simulink model "math_amp"  (Simulink 6.0)
settings: Solver=ode45  StartTime=0.0  StopTime=10.0  RelTol=1e-3
undefined symbols (not defined in the file or in its folder): dTypeID, Fs
libraries: dspsnks4 x2, rfmathmodels1 x1, dspmtrx3 x1, simulink x1
settings Model: Creator=ashivapr  LastModifiedBy=cvora  ExtModeAutoUpdateStatusClock=off  ProdHWDeviceType=Specified
settings DataIOCC: SaveOutput=off  SaveTime=off  SignalLoggingName=logsOut
settings DebuggingCC: CheckExecutionContextPreStartOutputMsg=on  CheckExecutionContextRuntimeOutputMsg=on  SolverPrmCheckMsg=none
settings HardwareCC: ProdHWDeviceType=Specified
settings ModelReferenceCC: UpdateModelReferenceTargets=IfOutOfDate
settings GRTTargetCC: LifeSpan=inf
settings SFSimCC: SFSimApplyToAllLibs=on  SFSimBuildMode=Incremental

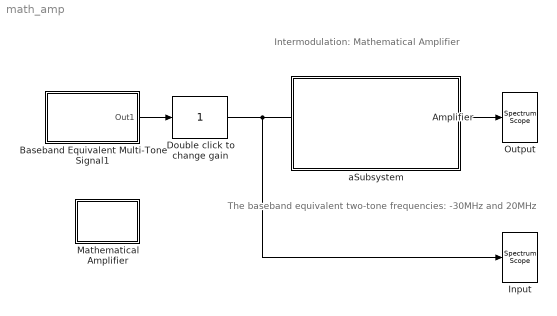
== system math_amp ==
  note: Intermodulation: Mathematical Amplifier
  note: The baseband equivalent
      |  two-tone frequencies:
      | -30MHz and 20MHz
  Amplifier : rfmathmodels1/Amplifier  model_select=Hyperbolic tangent  linGaindB=0  GindB=0  iip3=30  am2pm=0  amam=[2.1587 1.1517]  ampm=[4.0033 9.1040]  x=[8.1081 1.5413 6.5202 -0.0718]  y=[4.6645 2.0965 10.88 -0.003]  p=0.5  GoutdB=0  vsat=1  method_select=Noise figure  ntemp=290  nfigure=3.01  nfactor=2  seed=67987
  Baseband Equivalent Multi-Tone Signal1 : Subsystem  EnableExecutionContextPropagation=on  mask(Baseband Equivalent Multi-Tone Sine Wave){Fc=2.1e9, Frequency=[2.07e9 2.12e9], Amplitude=[0.01 0.005], Phase=[0 pi/4], SampleTime=3e-9, SamplesPerFrame=256}
      mask prompts: Fc "Center frequency (Hz)"; Frequency "Tone frequency (Hz):"; Amplitude "Tone amplitude:"; Phase "Tone phase offset (rad):"; SampleTime "Sample time:"; SamplesPerFrame "Samples per frame:"
      mask help:
      | Generate a baseband equivalent multi-tone complex sinusoid signal. The frequency of the output multi-tone signal is the difference between the Tone frequency and the Center frequency.
      |
      | The values specified here for the Center frequency and Sample time parameters should be equal to the values specified in the 'Input Port' block.
      mask init:
      | if ~isscalar(Fc)
      | 	error('Center frequency must be a scalar');
      | end
      | if ~isnumeric(Frequency)
      | 	error('Tone frequency must be a real vector');
      | end
      | if any(Frequency>=2*Fc)
      | 	error('Tone frequency is too large compared to the Center frequency');
      | end
      | 
      | Frequency = Frequency-Fc;
      mask Display:
      | plot(-0.5,-3,1.5,1,[0:0.005:1], [0.25*sin(2*pi*5*[0:0.005:1])+0.5*sin(2*pi*10*[0:0.005:1]) ]);
      | disp('\nMulti-Tone');
  Double click to change gain : simulink/Math Operations/Slider Gain  low=1  gain=1  high=10
  Input : dspsnks4/Spectrum Scope  ScopeProperties=off  Domain=Frequency  HorizSpan=1  UseBuffer=off  BufferSize=128  Overlap=64  inpFftLenInherit=off  FFTlength=1024  numAvg=20  DisplayProperties=on  AxisGrid=on  Memory=off  FrameNumber=off  AxisLegend=off  AxisZoom=off  OpenScopeAtSimStart=on  OpenScopeImmediately=off  FigPos=[6 311 333 250]  AxisProperties=off  XUnits=Hertz  XRange=[-Fs/2...Fs/2]  InheritXIncr=on  XIncr=1.0  XLabel=Samples  YUnits=dB  YLabel=Magnitude, dB  LineProperties=off
      settings: YMin=-162.913297942411  YMax=-10.4261857162777
  Mathematical Amplifier : Subsystem  EnableExecutionContextPropagation=on
      mask Display: disp('Info')
  Output : dspsnks4/Spectrum Scope  ScopeProperties=off  Domain=Frequency  HorizSpan=1  UseBuffer=off  BufferSize=128  Overlap=64  inpFftLenInherit=off  FFTlength=1024  numAvg=20  DisplayProperties=on  AxisGrid=on  Memory=off  FrameNumber=off  AxisLegend=off  AxisZoom=off  OpenScopeAtSimStart=on  OpenScopeImmediately=off  FigPos=[346 311 350 250]  AxisProperties=off  XUnits=Hertz  XRange=[-Fs/2...Fs/2]  InheritXIncr=on  XIncr=1.0  XLabel=Samples  YUnits=dB  YLabel=Magnitude, dB  LineProperties=off
      settings: YMin=-127.684741352242  YMax=8.6774665535425
  aSubsystem : Subsystem  EnableExecutionContextPropagation=on
      mask Display: disp('')
  wires:
  Baseband Equivalent Multi-Tone Signal1/1(Out1) -> Double click to change gain/1
  Amplifier/1 -> Output/1
  Double click to change gain/1 -> Input/1, Amplifier/1

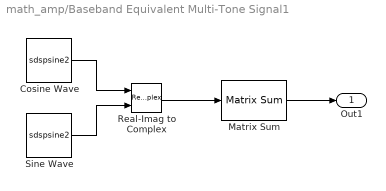
== system math_amp/Baseband Equivalent Multi-Tone Signal1 ==
  Cosine Wave : S-Function  AncestorBlock=dspsrcs4/Sine Wave  FunctionName=sdspsine2  Parameters=Amplitude,Frequency,Phase,SampleMode,OutComplex,CompMethod,SampleTime,SamplesPerFrame,ResetState,TableSize,isCustomFloat,isSigned,dTypeID,wordLength,fracBits  mask(Sine Wave){Amplitude=Amplitude, Frequency=Frequency, Phase=Phase+(pi/2), SampleMode=Discrete, OutComplex=Real, CompMethod=Trigonometric fcn, TableSize=Speed, SampleTime=SampleTime, SamplesPerFrame=SamplesPerFrame, additionalParams=off, allowOverrides=on, dataType=double, wordLen=16, udDataType=sfix(16), fracBitsMode=Best precision, numFracBits=15, ResetState=Restart at time zero}
      mask prompts: Frequency "Frequency (Hz):"; Phase "Phase offset (rad):"; SampleMode "Sample mode:"; OutComplex "Output complexity:"; CompMethod "Computation method:"; TableSize "Optimize table for:"; SampleTime "Sample time:"; SamplesPerFrame "Samples per frame:"; additionalParams "------- Show additional parameters --------"; allowOverrides "Allow overrides from DSP Fixed-Point Attributes blocks"; dataType "Output data type:"; wordLen "Word length:"; udDataType "User-defined data type (e.g. sfix(16), float('single')):"; fracBitsMode "Set fraction length in output to:"; numFracBits "Fraction length:"; ResetState "State when re-enabled:"
      mask help: Output samples of a sinusoid. To generate more than one sinusoid simultaneously, enter a vector of values for the amplitude, frequency, and phase parameters.
      mask init:
      | [x,y] = dspblksine('icon');
      | [dtInfo,dTypeID]=dspblksine('init');
      | isSigned=dtInfo.DataTypeIsSigned;
      | isCustomFloat=dtInfo.DataTypeIsCustomFloat;
      | wordLength=dtInfo.DataTypeWordLength;
      | fracBits=dtInfo.DataTypeFracOrMantBits;
      | dType=dataType;
      mask Help: web(dspbhelp);
      mask StyleString: edit,edit,edit,popup(Discrete|Continuous),popup(Real|Complex),popup(Trigonometric fcn|Table lookup|Differential),popup(Speed|Memory),edit,edit,checkbox,checkbox,popup(double|single|Fixed-point|User-defined|Inherit via back propagation),edit,edit,popup(Best precision|User-defined),edit,popup(Restart at time zero|Catch up to simulation time)
      mask CallbackString: |||dspblksine;||dspblksine;||||dspblksine|dspblksine|dspblksine||dspblksine|dspblksine||
      mask Display:
      | plot(x,y)
      | text(3.25,.75,'DSP');
  Matrix Sum : dspmtrx3/Matrix Sum  Dim=Rows  roundingMode=Floor  overflowMode=off
  Real-Imag to Complex : RealImagToComplex
  Sine Wave : S-Function  AncestorBlock=dspsrcs4/Sine Wave  FunctionName=sdspsine2  Parameters=Amplitude,Frequency,Phase,SampleMode,OutComplex,CompMethod,SampleTime,SamplesPerFrame,ResetState,TableSize,isCustomFloat,isSigned,dTypeID,wordLength,fracBits  mask(Sine Wave){Amplitude=Amplitude, Frequency=Frequency, Phase=Phase, SampleMode=Discrete, OutComplex=Real, CompMethod=Trigonometric fcn, TableSize=Speed, SampleTime=SampleTime, SamplesPerFrame=SamplesPerFrame, additionalParams=off, allowOverrides=on, dataType=double, wordLen=16, udDataType=sfix(16), fracBitsMode=Best precision, numFracBits=15, ResetState=Restart at time zero}
      mask prompts: Frequency "Frequency (Hz):"; Phase "Phase offset (rad):"; SampleMode "Sample mode:"; OutComplex "Output complexity:"; CompMethod "Computation method:"; TableSize "Optimize table for:"; SampleTime "Sample time:"; SamplesPerFrame "Samples per frame:"; additionalParams "------- Show additional parameters --------"; allowOverrides "Allow overrides from DSP Fixed-Point Attributes blocks"; dataType "Output data type:"; wordLen "Word length:"; udDataType "User-defined data type (e.g. sfix(16), float('single')):"; fracBitsMode "Set fraction length in output to:"; numFracBits "Fraction length:"; ResetState "State when re-enabled:"
      mask help: Output samples of a sinusoid. To generate more than one sinusoid simultaneously, enter a vector of values for the amplitude, frequency, and phase parameters.
      mask init: same as math_amp/Baseband Equivalent Multi-Tone Signal1/Cosine Wave
      mask Help: web(dspbhelp);
      mask StyleString: edit,edit,edit,popup(Discrete|Continuous),popup(Real|Complex),popup(Trigonometric fcn|Table lookup|Differential),popup(Speed|Memory),edit,edit,checkbox,checkbox,popup(double|single|Fixed-point|User-defined|Inherit via back propagation),edit,edit,popup(Best precision|User-defined),edit,popup(Restart at time zero|Catch up to simulation time)
      mask CallbackString: |||dspblksine;||dspblksine;||||dspblksine|dspblksine|dspblksine||dspblksine|dspblksine||
      mask Display:
      | plot(x,y)
      | text(3.25,.75,'DSP');
  Out1 : Outport
  wires:
  Matrix Sum/1 -> Out1/1
  Cosine Wave/1 -> Real-Imag to Complex/1
  Sine Wave/1 -> Real-Imag to Complex/2
  Real-Imag to Complex/1 -> Matrix Sum/1

== system math_amp/Mathematical Amplifier ==
  note: Intermodulation: Mathematical Amplifier
      |
      | The 'Mathematical Amplifier' block is
      | a complex  baseband model and not frequency-dependent.
      |
      | To view the intermodulation performance at the output,
      | double click the 'Slider Gain' block and change the gain
      | while the model is running.
      |
      | To compare with the intermodulation of the physical
      | amplifier, simulate the demo:
      | Comparison of Amplifiers: Linear vs Nonlinear.

== system math_amp/aSubsystem ==
